simulink model "quadrotor_Simulink_Main"  (R2024b)
settings: Solver=VariableStepAuto  StartTime=0.0  StopTime=30  RelTol=1e-3
values from neighbouring files (symbols this model uses):
  b = 3.13*10^(-5)    (= 3.13e-05)    [quad_model_sim.m]
  d = 7.5*10^(-7)    (= 7.5e-07)    [quad_model_sim.m]
  g = 9.81    [quad_model_sim.m]
  Ir = 6.5*10^(-5)    (= 6.5e-05)    [quad_model_sim.m]
  Ix = 7.5*10^(-3)    (= 0.0075)    [quad_model_sim.m]
  Iy = 7.5*10^(-3)    (= 0.0075)    [quad_model_sim.m]
  Iz = 1.3*10^(-2)    (= 0.013)    [quad_model_sim.m]
  l = 0.23    [quad_model_sim.m]
  m = 0.65    [quad_model_sim.m]
libraries: slpidlib x11, simulink_extras x6, sim3dlib x1, uavsim3dlib x1
(part 2 of 2)

== matlab function quadrotor_Simulink_Main/POSITION CONTROLLER/Trajectory Generation Function ==
  data: t input; x_d output; y_d output; z_d output; psi_d output
function [x_d, y_d, z_d, psi_d] = fcn(t)

% if t < 10
%     % Climb straight up to 50m
%     x_d = 0;   y_d = 0;   z_d = 5*t;  psi_d = 0;
% elseif t < 20
%     % Pitch forward: move 20m in X
%     x_d = 20;  y_d = 0;   z_d = 50;   psi_d = 0;
% else
%     % Roll right: move 20m in Y
%     x_d = 20;  y_d = 20;  z_d = 50;   psi_d = 0;
% end

x_d = cos(0.2*t);
y_d = sin(0.2*t);
z_d = 10*t;
psi_d = sin(t);

end

% x_d = cos(0.5*t);
% y_d = sin(0.5*t);
% z_d = 0.5*t;
% psi_d = sin(t);

== matlab function quadrotor_Simulink_Main/Rotational Dynamics/function to calculate Omega ==
  data: T input; T_phi input; Omega output; T_theta input; T_psi input; b input; l input; d input
function Omega = fcn(T, T_phi, T_theta, T_psi, b, l, d)

U1 = T/b;
U2 = T_phi/(l*b);
U3 = T_theta/(l*b);
U4 = T_psi/d;

omega_3 = sqrt(max(0,(U1 + U4 + 2*U2)/4));
omega_1 = sqrt(max(0,(U1 + U4 - 2*U2)/4));
omega_4 = sqrt(max(0,(U1 - U4 + 2*U3)/4));
omega_2 = sqrt(max(0,(U1 - U4 - 2*U3)/4));

Omega = omega_1 - omega_2 + omega_3 - omega_4;
end

== matlab function quadrotor_Simulink_Main/POSITION CONTROLLER/MATLAB Function1 ==
  data: T_x input; T_y input; Phi_desired output; T_z input; psi_d input; Theta_desired output; Thrust_desired output
function [Phi_desired, Theta_desired, Thrust_desired] = fcn(T_x, T_y, T_z, psi_d)

Phi_desired   =  ((T_x*sin(psi_d)- T_y*cos(psi_d))/T_z);
Theta_desired =  ((T_x*cos(psi_d)+ T_y*sin(psi_d))/(cos(Phi_desired)*T_z));
Thrust_desired        =  T_z;

Phi_desired = max(Phi_desired,-pi/6);
Phi_desired = min(Phi_desired, pi/6);

Theta_desired = max(Theta_desired,-pi/6);
Theta_desired = min(Theta_desired, pi/6);
